simulink model "renewable_energy_assignment1_t1"  (R2024b)
settings: Solver=VariableStepAuto  StartTime=0.0  StopTime=100  RelTol=1e-3
settings Model: Creator=zeyneptutumlu
settings ModelReferenceCC: UpdateModelReferenceTargets=IfOutOfDate
settings ConfigComp: CovBoundaryAbsTol=1.0e-5

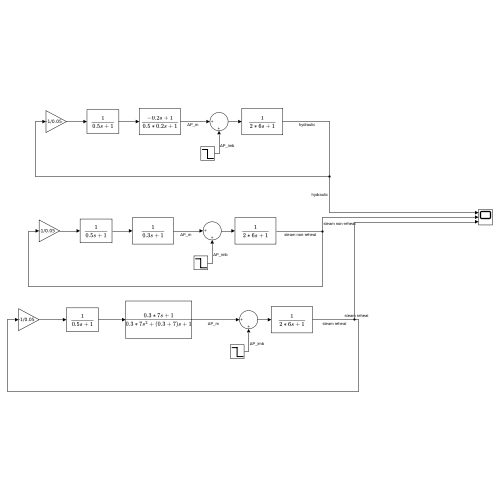
[thumbnail: Simulink's stored preview of the top-level diagram]
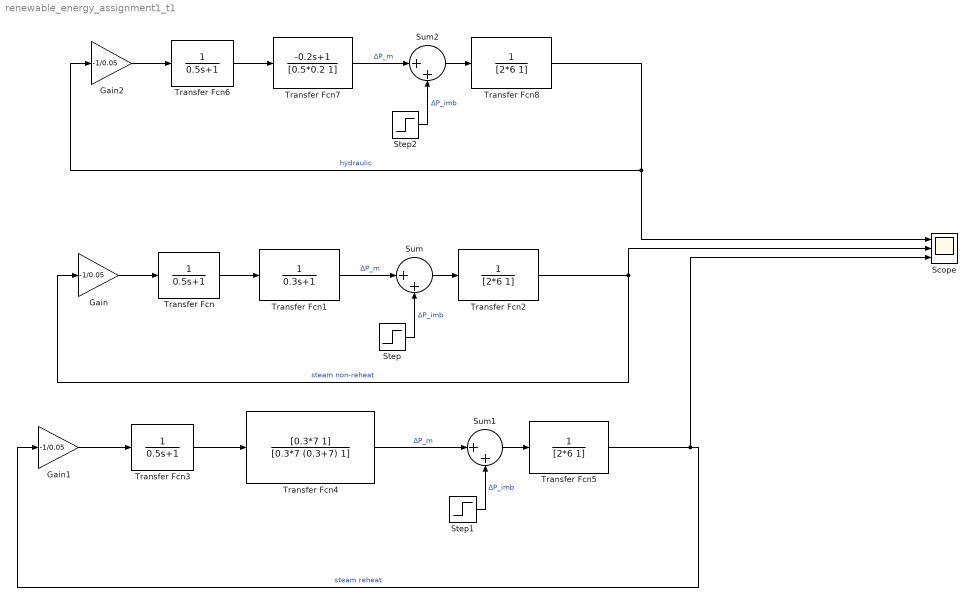
== system renewable_energy_assignment1_t1 ==
  Gain : Gain  Gain=-1/0.05
  Gain1 : Gain  Gain=-1/0.05
  Gain2 : Gain  Gain=-1/0.05
  Scope : Scope  NumInputPorts=3
  Step : Step  After=-0.1  SampleTime=0
  Step1 : Step  After=-0.1  SampleTime=0
  Step2 : Step  After=-0.1  SampleTime=0
  Sum : Sum  Inputs=|++
  Sum1 : Sum  Inputs=|++
  Sum2 : Sum  Inputs=|++
  Transfer Fcn : TransferFcn  Denominator=[0.5 1]
  Transfer Fcn1 : TransferFcn  Denominator=[0.3 1]
  Transfer Fcn2 : TransferFcn  Denominator=[2*6 1]
  Transfer Fcn3 : TransferFcn  Denominator=[0.5 1]
  Transfer Fcn4 : TransferFcn  Numerator=[0.3*7 1]  Denominator=[0.3*7 (0.3+7) 1]
  Transfer Fcn5 : TransferFcn  Denominator=[2*6 1]
  Transfer Fcn6 : TransferFcn  Denominator=[0.5 1]
  Transfer Fcn7 : TransferFcn  Numerator=[-0.2 1]  Denominator=[0.5*0.2 1]
  Transfer Fcn8 : TransferFcn  Denominator=[2*6 1]
  wires:
  Sum/1 -> Transfer Fcn2/1
  Transfer Fcn2/1 -> Scope/2, Gain/1  "steam non-reheat"
  Gain/1 -> Transfer Fcn/1
  Transfer Fcn1/1 -> Sum/1  "ΔP_m"
  Step/1 -> Sum/2  "ΔP_imb"
  Transfer Fcn/1 -> Transfer Fcn1/1
  Step1/1 -> Sum1/2  "ΔP_imb"
  Transfer Fcn5/1 -> Gain1/1, Scope/3  "steam reheat"
  Gain1/1 -> Transfer Fcn3/1
  Transfer Fcn4/1 -> Sum1/1  "ΔP_m"
  Sum1/1 -> Transfer Fcn5/1
  Transfer Fcn3/1 -> Transfer Fcn4/1
  Sum2/1 -> Transfer Fcn8/1
  Transfer Fcn8/1 -> Scope/1, Gain2/1  "hydraulic"
  Gain2/1 -> Transfer Fcn6/1
  Transfer Fcn7/1 -> Sum2/1  "ΔP_m"
  Step2/1 -> Sum2/2  "ΔP_imb"
  Transfer Fcn6/1 -> Transfer Fcn7/1
